simulink model "desperate_measures"  (R2021b)
settings: Solver=VariableStepAuto  StartTime=0.0  StopTime=10.0  RelTol=1e-3
libraries: simulink x1, mpclib x1
settings Model: Creator=luismiguelmartinezgomez  LastModifiedBy=luismiguelmartinezgomez

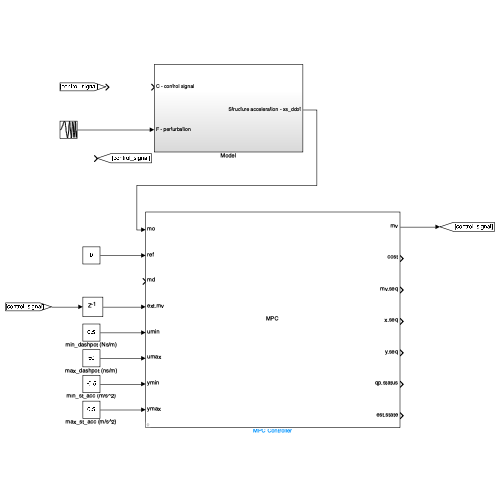
[thumbnail: Simulink's stored preview of the top-level diagram]
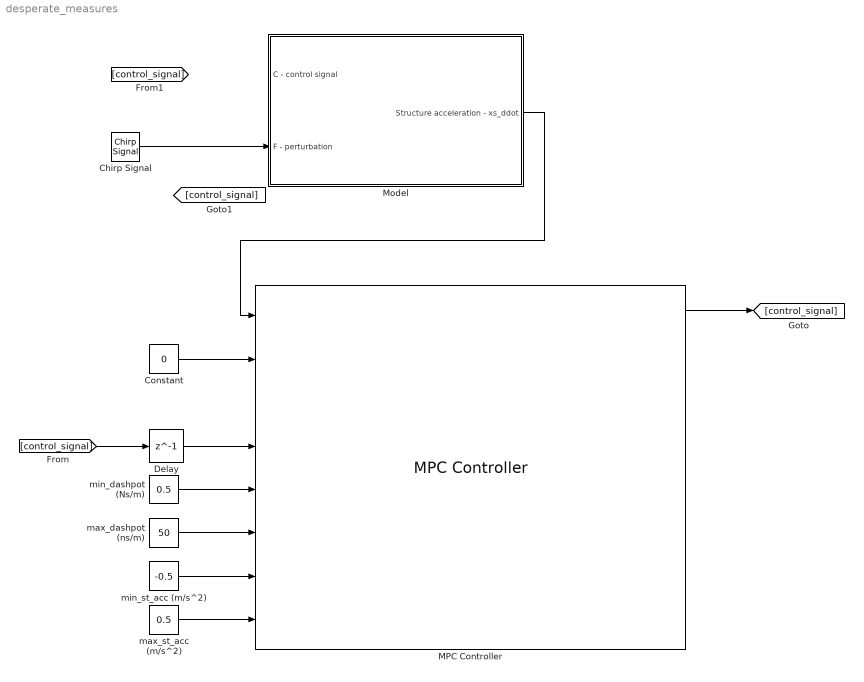
== system desperate_measures ==
  Chirp Signal : simulink/Sources/Chirp Signal  f1=0.1  T=100  f2=1
  Constant : Constant  Value=0
  Delay : Delay  DelayLength=1
  MPC Controller : mpclib/MPC Controller  SCDEnableBlockLinearizationSpecification=on  is_multiple=0  enable_value=0  return_u0=off  updateMPCinCallerWorkspace=on  md_inport=on  mv_inport=on  uref_inport=off  return_cost=on  return_mvseq=on  return_qpstatus=on  return_xseq=on  return_state=on  return_ovseq=on  state_inport=off  umin_inport=on  umax_inport=on  ymin_inport=on  ymax_inport=on  cc_inport=off  ywt_inport=off  uwt_inport=off  duwt_inport=off  rhoeps_inport=off  pm_inport=off  MaximumP=10  HorizonChoice=FixedHorizon  n_ts=1  n_p=10  n_mv=1  n_md=1  n_ud=0  n_mo=1  n_uo=0  BlockDataType=double  SampleTimeInherited=off  switch_inport=off
  Model : Subsystem
  max_dashpot (ns/m) : Constant  Value=50
  max_st_acc (m/s^2) : Constant  Value=0.5
  min_dashpot (Ns/m) : Constant  Value=0.5
  min_st_acc (m/s^2) : Constant  Value=-0.5
  wires:
  Model/1(Structure acceleration - xs_ddot) -> MPC Controller/1
  Constant/1 -> MPC Controller/2
  Delay/1 -> MPC Controller/4
  MPC Controller/1 -> [control_signal]
  [control_signal] -> Delay/1
  min_st_acc (m/s^2)/1 -> MPC Controller/7
  max_st_acc (m/s^2)/1 -> MPC Controller/8
  max_dashpot (ns/m)/1 -> MPC Controller/6
  min_dashpot (Ns/m)/1 -> MPC Controller/5
  Chirp Signal/1 -> Model/2(F - perturbation)

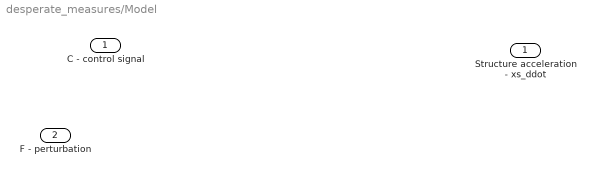
== system desperate_measures/Model ==
  C - control signal : Inport
  F - perturbation : Inport  Port=2
  Structure acceleration - xs_ddot : Outport
  wires:
  ? -> Structure acceleration - xs_ddot/1
